simulink model "sampleModel1833"  (R2023a)
settings: Solver=VariableStepAuto  StartTime=0.0  StopTime=10.0  RelTol=1e-3
libraries: simulink x2, hdlsllib x2
settings Model: Creator=user1  LastModifiedBy=user1

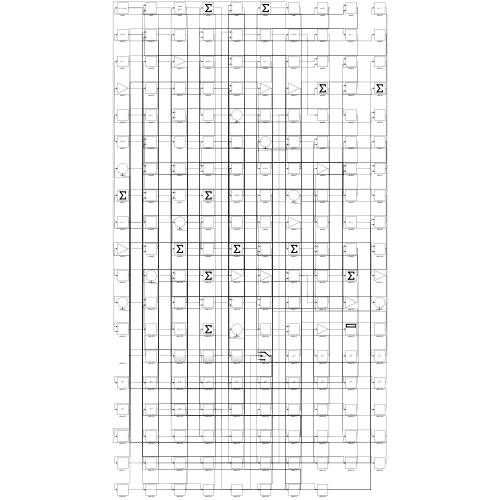
[thumbnail: Simulink's stored preview of the top-level diagram]
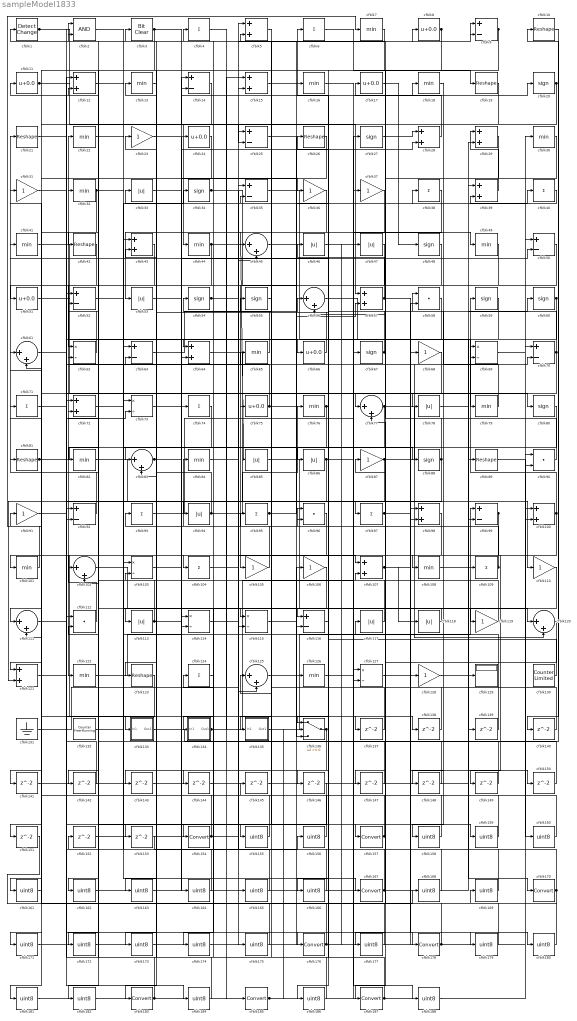
== system sampleModel1833 ==
  cfblk1 : simulink/Logic and Bit Operations/Detect Change  vinit=0  OutDataTypeStr=boolean
      settings: LibrarySourceBlock=|
      | hdlsllib/Logic and Bit
      | Operations/Detect
      | Change
  cfblk{10,19,21,26,42,81,89,123} (8 alike) : Reshape
  cfblk{5,12,15,28..29,39,43,57,64,72,98,100,107,121} (14 alike) : Sum
  cfblk{7,13,16,18,22,30,32,41,44,49,65,76,79,82,84,101,108,122,126} (19 alike) : MinMax
  cfblk{45,56,61,77,83,102,111,120,125} (9 alike) : Sum  Inputs=|++
  cfblk{62,69,73,103,114..115,127} (7 alike) : Product  Inputs=*/  RndMeth=Zero  SaturateOnIntegerOverflow=on
  cfblk{4,6,38,40,71,74,93,95,97,104,109,124} (12 alike) : Sum  Inputs=+
  cfblk{23,31,36..37,68,87,91,105..106,110,119,128} (12 alike) : Gain
  cfblk{8,11,17,24,51,66,75} (7 alike) : Bias  Bias=0.0  SaturateOnIntegerOverflow=off
  cfblk{58,90,96,112} (4 alike) : DotProduct  OutDataTypeStr=Inherit: Inherit via internal rule
  cfblk{33,46..47,53,78,85..86,94,113,117..118} (11 alike) : Abs  SaturateOnIntegerOverflow=off
  cfblk{9,14,25,35,50,52,63,70,92,99,116} (11 alike) : Sum  Inputs=+-
  cfblk129 : Display
  cfblk130 : hdlsllib/Sources/Counter Limited  uplimit=7  tsamp=-1
  cfblk131 : Ground
  cfblk132 : hdlsllib/Sources/Counter Free-Running  NumBits=16  tsamp=-1
  cfblk133 : Subsystem
      settings: LibrarySourceBlock=|
      | hdlsllib/Ports &
      | Subsystems/Subsystem
  cfblk134 : Subsystem
      settings: LibrarySourceBlock=|
      | hdlsllib/Ports &
      | Subsystems/Subsystem
  cfblk135 : Subsystem
      settings: LibrarySourceBlock=|
      | hdlsllib/Ports &
      | Subsystems/Subsystem
  cfblk136 : Switch  SaturateOnIntegerOverflow=off  InputSameDT=off
  cfblk{137..153} (17 alike) : Delay  SampleTime=1
  cfblk{154,157,167,170,176,178,183,185,187} (9 alike) : DataTypeConversion  SaturateOnIntegerOverflow=off  RndMeth=Floor
  cfblk{155..156,158..166,168..169,171..175,177,179..182,184,186,188} (26 alike) : DataTypeConversion  OutDataTypeStr=uint8  SaturateOnIntegerOverflow=off  RndMeth=Floor
  cfblk2 : Logic  AllPortsSameDT=off  OutDataTypeStr=boolean
  cfblk{20,27,34,48,54..55,59..60,67,80,88} (11 alike) : Signum
  cfblk3 : simulink/Logic and Bit Operations/Bit Clear  iBit=0
      settings: LibrarySourceBlock=|
      | hdlsllib/Logic and Bit
      | Operations/Bit Clear
  wires:
  cfblk100/1 -> cfblk59/1, cfblk115/2, cfblk149/1
  cfblk60/1 -> cfblk64/2, cfblk163/1
  cfblk92/1 -> cfblk21/1
  cfblk17/1 -> cfblk48/1
  cfblk98/1 -> cfblk104/1
  cfblk102/1 -> cfblk116/1
  cfblk67/1 -> cfblk33/1, cfblk64/1
  cfblk64/1 -> cfblk110/1
  cfblk81/1 -> cfblk133/1(In1), cfblk73/2
  cfblk19/1 -> cfblk44/1
  cfblk47/1 -> cfblk105/1
  cfblk96/1 -> cfblk122/1
  cfblk112/1 -> cfblk22/1
  cfblk135/1(Out1) -> cfblk99/1
  cfblk51/1 -> cfblk66/1
  cfblk133/1(Out1) -> cfblk10/1
  cfblk11/1 -> cfblk57/1, cfblk78/1
  cfblk12/1 -> cfblk167/1
  cfblk85/1 -> cfblk120/1
  cfblk7/1 -> cfblk82/1
  cfblk44/1 -> cfblk85/1, cfblk171/1
  cfblk131/1 -> cfblk25/1
  cfblk70/1 -> cfblk41/1, cfblk135/1(In1)
  cfblk77/1 -> cfblk120/2, cfblk123/1
  cfblk15/1 -> cfblk6/1
  cfblk29/1 -> cfblk108/1
  cfblk105/1 -> cfblk93/1
  cfblk65/1 -> cfblk54/1
  cfblk104/1 -> cfblk18/1
  cfblk28/1 -> cfblk17/1
  cfblk125/1 -> cfblk68/1
  cfblk93/1 -> cfblk37/1
  cfblk118/1 -> cfblk113/1
  cfblk35/1 -> cfblk109/1
  cfblk27/1 -> cfblk28/1
  cfblk24/1 -> cfblk121/1
  cfblk14/1 -> cfblk51/1
  cfblk94/1 -> cfblk76/1, cfblk62/2
  cfblk45/1 -> cfblk79/1
  cfblk58/1 -> cfblk92/2
  cfblk26/1 -> cfblk111/1
  cfblk82/1 -> cfblk114/1
  cfblk88/1 -> cfblk2/2, cfblk181/1
  cfblk73/1 -> cfblk28/2
  cfblk25/1 -> cfblk116/2
  cfblk126/1 -> cfblk38/1
  cfblk130/1 -> cfblk96/1
  cfblk134/1(Out1) -> cfblk27/1, cfblk15/1
  cfblk71/1 -> cfblk176/1
  cfblk23/1 -> cfblk157/1
  cfblk46/1 -> cfblk49/1
  cfblk13/1 -> cfblk183/1
  cfblk41/1 -> cfblk89/1
  cfblk110/1 -> cfblk134/1(In1)
  cfblk66/1 -> cfblk3/1
  cfblk84/1 -> cfblk9/1
  cfblk32/1 -> cfblk119/1, cfblk141/1
  cfblk1/1 -> cfblk67/1, cfblk100/2
  cfblk101/1 -> cfblk7/1
  cfblk42/1 -> cfblk62/1
  cfblk119/1 -> cfblk81/1
  cfblk37/1 -> cfblk53/1
  cfblk128/1 -> cfblk170/1
  cfblk80/1 -> cfblk136/1
  cfblk132/1 -> cfblk34/1
  cfblk3/1 -> cfblk111/2, cfblk25/2
  cfblk113/1 -> cfblk14/1, cfblk11/1
  cfblk76/1 -> cfblk114/2, cfblk166/1
  cfblk109/1 -> cfblk84/1, cfblk43/2
  cfblk87/1 -> cfblk39/1, cfblk121/2
  cfblk75/1 -> cfblk2/1, cfblk80/1
  cfblk69/1 -> cfblk50/1
  cfblk91/1 -> cfblk65/1
  cfblk34/1 -> cfblk126/1, cfblk125/2
  cfblk95/1 -> cfblk9/2, cfblk57/2
  cfblk62/1 -> cfblk32/1
  cfblk4/1 -> cfblk185/1
  cfblk8/1 -> cfblk14/2, cfblk153/1
  cfblk9/1 -> cfblk97/1, cfblk146/1
  cfblk20/1 -> cfblk42/1, cfblk75/1
  cfblk57/1 -> cfblk46/1, cfblk150/1
  cfblk53/1 -> cfblk20/1
  cfblk30/1 -> cfblk187/1
  cfblk22/1 -> cfblk86/1
  cfblk136/1 -> cfblk143/1, cfblk144/1
  cfblk115/1 -> cfblk136/3
  cfblk33/1 -> cfblk36/1
  cfblk49/1 -> cfblk77/1
  cfblk6/1 -> cfblk19/1
  cfblk108/1 -> cfblk60/1
  cfblk99/1 -> cfblk102/1, cfblk101/1
  cfblk55/1 -> cfblk115/1
  cfblk83/1 -> cfblk50/2, cfblk69/1
  cfblk97/1 -> cfblk69/2, cfblk147/1
  cfblk79/1 -> cfblk58/1
  cfblk5/1 -> cfblk45/1
  cfblk116/1 -> cfblk16/1
  cfblk40/1 -> cfblk39/2
  cfblk117/1 -> cfblk56/1
  cfblk38/1 -> cfblk83/1
  cfblk72/1 -> cfblk154/1
  cfblk54/1 -> cfblk107/1, cfblk8/1
  cfblk56/1 -> cfblk129/1
  cfblk2/1 -> cfblk43/1
  cfblk63/1 -> cfblk40/1
  cfblk78/1 -> cfblk70/2
  cfblk52/1 -> cfblk88/1
  cfblk90/1 -> cfblk56/2
  cfblk86/1 -> cfblk94/1, cfblk138/1
  cfblk31/1 -> cfblk178/1
  cfblk39/1 -> cfblk29/1
  cfblk122/1 -> cfblk24/1
  cfblk107/1 -> cfblk98/2, cfblk118/1, cfblk87/1
  cfblk121/1 -> cfblk137/1
  cfblk137/1 -> cfblk1/1
  cfblk138/1 -> cfblk107/2
  cfblk139/1 -> cfblk63/1
  cfblk10/1 -> cfblk140/1
  cfblk140/1 -> cfblk98/1
  cfblk141/1 -> cfblk15/2
  cfblk43/1 -> cfblk142/1
  cfblk142/1 -> cfblk92/1
  cfblk143/1 -> cfblk99/2
  cfblk144/1 -> cfblk29/2
  cfblk145/1 -> cfblk58/2
  cfblk147/1 -> cfblk102/2
  cfblk59/1 -> cfblk148/1
  cfblk148/1 -> cfblk112/2
  cfblk149/1 -> cfblk5/2
  cfblk150/1 -> cfblk52/2
  cfblk68/1 -> cfblk151/1
  cfblk152/1 -> cfblk45/2
  cfblk154/1 -> cfblk91/1, cfblk165/1
  cfblk36/1 -> cfblk155/1
  cfblk155/1 -> cfblk72/1
  cfblk153/1 -> cfblk156/1
  cfblk156/1 -> cfblk72/2
  cfblk157/1 -> cfblk83/2, cfblk5/1
  cfblk18/1 -> cfblk158/1
  cfblk158/1 -> cfblk23/1
  cfblk61/1 -> cfblk159/1
  cfblk159/1 -> cfblk96/2
  cfblk89/1 -> cfblk160/1
  cfblk160/1 -> cfblk61/1
  cfblk123/1 -> cfblk161/1
  cfblk161/1 -> cfblk61/2
  cfblk74/1 -> cfblk162/1
  cfblk162/1 -> cfblk139/1
  cfblk163/1 -> cfblk74/1
  cfblk103/1 -> cfblk164/1
  cfblk164/1 -> cfblk63/2
  cfblk165/1 -> cfblk103/1
  cfblk166/1 -> cfblk103/2
  cfblk167/1 -> cfblk35/1, cfblk125/1, cfblk95/1, cfblk73/1
  cfblk151/1 -> cfblk168/1
  cfblk168/1 -> cfblk12/1
  cfblk169/1 -> cfblk12/2
  cfblk170/1 -> cfblk169/1, cfblk55/1
  cfblk171/1 -> cfblk128/1
  cfblk106/1 -> cfblk172/1
  cfblk172/1 -> cfblk90/1
  cfblk48/1 -> cfblk173/1
  cfblk173/1 -> cfblk106/1
  cfblk124/1 -> cfblk174/1
  cfblk174/1 -> cfblk90/2
  cfblk114/1 -> cfblk175/1
  cfblk175/1 -> cfblk124/1
  cfblk176/1 -> cfblk145/1, cfblk47/1
  cfblk120/1 -> cfblk177/1
  cfblk177/1 -> cfblk71/1
  cfblk178/1 -> cfblk117/1, cfblk77/2
  cfblk111/1 -> cfblk179/1
  cfblk179/1 -> cfblk31/1
  cfblk127/1 -> cfblk180/1
  cfblk180/1 -> cfblk112/1
  cfblk181/1 -> cfblk127/1
  cfblk146/1 -> cfblk182/1
  cfblk182/1 -> cfblk127/2
  cfblk183/1 -> cfblk152/1, cfblk70/1
  cfblk21/1 -> cfblk184/1
  cfblk184/1 -> cfblk13/1
  cfblk185/1 -> cfblk100/1, cfblk136/2
  cfblk50/1 -> cfblk186/1
  cfblk186/1 -> cfblk4/1
  cfblk187/1 -> cfblk35/2, cfblk26/1, cfblk52/1
  cfblk16/1 -> cfblk188/1
  cfblk188/1 -> cfblk30/1

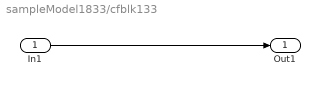
== system sampleModel1833/cfblk133 ==
  In1 : Inport
  Out1 : Outport
  wires:
  In1/1 -> Out1/1

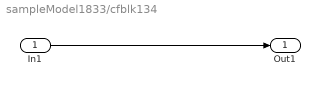
== system sampleModel1833/cfblk134 ==
  In1 : Inport
  Out1 : Outport
  wires:
  In1/1 -> Out1/1

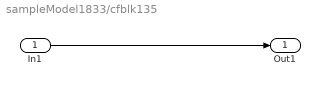
== system sampleModel1833/cfblk135 ==
  In1 : Inport
  Out1 : Outport
  wires:
  In1/1 -> Out1/1
